simulink model "example1"  (R2015b)
settings: Solver=VariableStepAuto  StartTime=0.0  StopTime=100  RelTol=1e-3
undefined symbols (not defined in the file): b, k, M
settings Model: Creator=pk  LastModifiedBy=pk

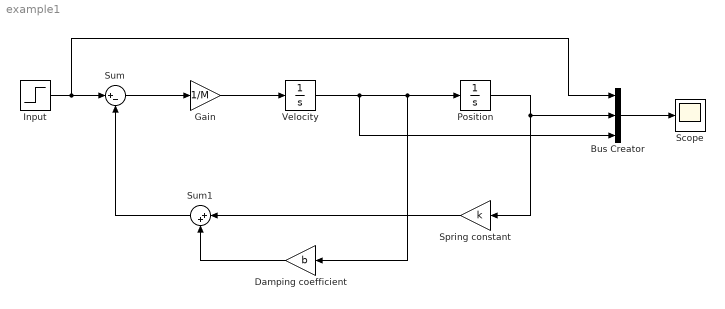
== system example1 ==
  Bus Creator : BusCreator  Inputs=3
  Damping coefficient : Gain  Gain=b
  Gain : Gain  Gain=1/M
  Input : Step  SampleTime=0
  Position : Integrator
  Scope : Scope
  Spring constant : Gain  Gain=k
  Sum : Sum  Inputs=|+-
  Sum1 : Sum  Inputs=|++
  Velocity : Integrator
  wires:
  Input/1 -> Bus Creator/1, Sum/1
  Sum/1 -> Gain/1
  Gain/1 -> Velocity/1
  Velocity/1 -> Bus Creator/3, Damping coefficient/1, Position/1
  Sum1/1 -> Sum/2
  Damping coefficient/1 -> Sum1/2
  Spring constant/1 -> Sum1/1
  Position/1 -> Spring constant/1, Bus Creator/2
  Bus Creator/1 -> Scope/1
